simulink model "Model_01"  (R2014a)
settings: Solver=ode45  StartTime=0.0  StopTime=10.0  RelTol=1e-3
model workspace: external: MATLAB File C:\Users\Iseberg\Documents\MATLAB\Init_Model_01.m (data not in the file)
values from neighbouring files (symbols this model uses):
  e_force_x = 0    [Init_Model_01.m]    (also in Init_Model_02_Simulink.m)
  e_force_y = 0    [Init_Model_01.m]    (also in Init_Model_02_Simulink.m)
  e_force_z = 0    [Init_Model_01.m]    (also in Init_Model_02_Simulink.m)
  ita = [0.12;0.05;-0.15;0.98]    [Init_Model_01.m]    (also in Init_Model_02_Simulink.m)
  J_k = J    [Init_Model_01.m]
  om_x_0 = 0    [Init_Model_01.m]    (also in Init_Model_02_Simulink.m)
  om_y_0 = 0    [Init_Model_01.m]    (also in Init_Model_02_Simulink.m)
  om_z_0 = 0    [Init_Model_01.m]    (also in Init_Model_02_Simulink.m)
  p_x = (i_yy - i_zz)/i_xx    (= 0.75)    [Init_Model_01.m]    (also in Init_Model_02_Simulink.m)
  p_x_0 = p_x    (= 0.75)    [Init_Model_01.m]    (also in Init_Model_02_Simulink.m = 2)
  p_y = (i_zz - i_xx)/i_yy    (= 0.125)    [Init_Model_01.m]    (also in Init_Model_02_Simulink.m)
  p_y_0 = p_y    (= 0.125)    [Init_Model_01.m]    (also in Init_Model_02_Simulink.m = -0.5)
  p_z = (i_xx - i_yy)/i_zz    (= -0.8)    [Init_Model_01.m]    (also in Init_Model_02_Simulink.m)
  p_z_0 = p_z    (= -0.8)    [Init_Model_01.m]    (also in Init_Model_02_Simulink.m = -2)
  q_0_0 = 1    [Init_Model_01.m]    (also in Init_Model_02_Simulink.m)
  q_1_0 = 0    [Init_Model_01.m]    (also in Init_Model_02_Simulink.m)
  q_2_0 = 0    [Init_Model_01.m]    (also in Init_Model_02_Simulink.m)
  q_3_0 = 0    [Init_Model_01.m]    (also in Init_Model_02_Simulink.m)
  r_dot_x_0 = 0    [Init_Model_01.m]    (also in Init_Model_02_Simulink.m)
  r_dot_y_0 = 0    [Init_Model_01.m]    (also in Init_Model_02_Simulink.m)
  r_dot_z_0 = 0    [Init_Model_01.m]    (also in Init_Model_02_Simulink.m)
  r_x_0 = 0    [Init_Model_01.m]    (also in Init_Model_02_Simulink.m)
  r_y_0 = 0    [Init_Model_01.m]    (also in Init_Model_02_Simulink.m)
  r_z_0 = 0    [Init_Model_01.m]    (also in Init_Model_02_Simulink.m)
  rho = [0.2;0.1;0.05]    [Init_Model_01.m]    (also in Init_Model_02_Simulink.m; quatErrorTest.m = fn_CrossTensor([a_g;2],0)*q_ref)
  sig_p = 1e-4    (= 0.0001)    [Init_Model_01.m]    (also in Init_Model_02_Simulink.m)
  sig_tau = 2.5e-5    (= 2.5e-05)    [Init_Model_01.m]    (also in Init_Model_02_Simulink.m)
  sig_theta = 1e-4    (= 0.0001)    [Init_Model_01.m]    (also in Init_Model_02_Simulink.m = 1e-06)
  tau_1 = 0    [Init_Model_01.m]    (also in Init_Model_02_Simulink.m)
  tau_2 = 0    [Init_Model_01.m]    (also in Init_Model_02_Simulink.m)
  tau_3 = 0    [Init_Model_01.m]    (also in Init_Model_02_Simulink.m)
undefined symbols (not defined in the file or in its folder): DiscIntNeverNeededParam
settings Model: Creator=Iseberg  LastModifiedBy=Iseberg

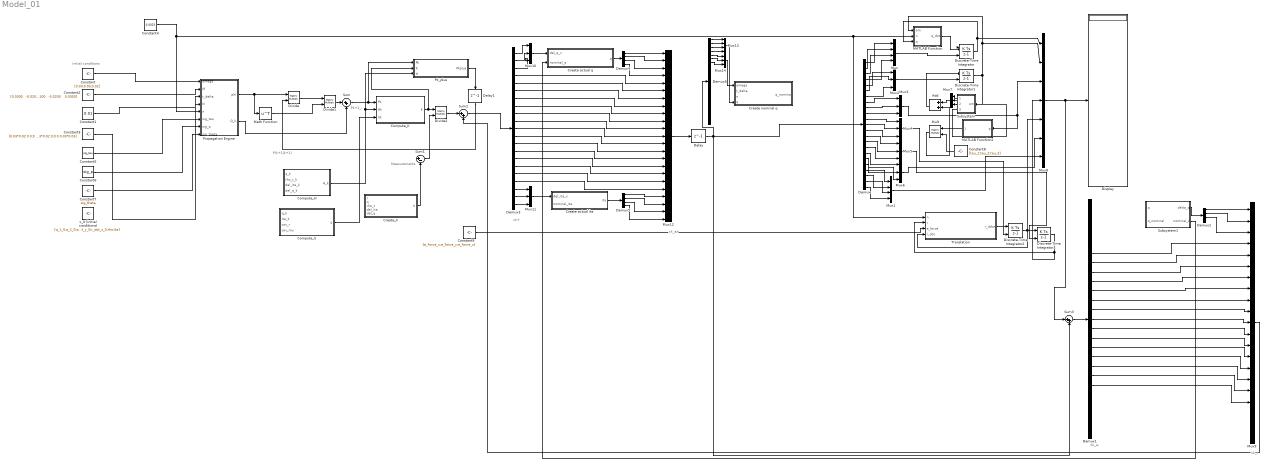
== system Model_01 ==
  note: initial conditions
  note: Pk+1_-
  note: xk_-
  note: xk_a-
  note: xk_a+
  note: xk+
  note: Measurements
  note: P(k+1|k+1)
  Add : Sum
  Compute_H : Subsystem
  Compute_K : MATLAB Function  TreatAsAtomicUnit=on
  Compute_S : MATLAB Function  TreatAsAtomicUnit=on
  Constant : Constant  Value=[0.03;0.03;0.02]
  Constant1 : Constant  Value=0.01
  Constant2 : Constant  Value="[0.0300   -0.0200    0.0100;-0.0200    0.0200   -0.0100;0.0100   -0.0200    0.0300]"
  Constant3 : Constant  Value=[0.03*0.02 0 0;0 0.03*0.02 0;0 0 0.03*0.03]
  Constant4 : Constant  Value=0.0023
  Constant5 : Constant  Value=sig_tau
  Constant6 : Constant  Value=sig_p
  Constant7 : Constant  Value=sig_theta
  Constant8 : Constant  Value=[tau_1;tau_2;tau_3]
  Constant9 : Constant  Value=[e_force_x;e_force_y;e_force_z]
  Create actual ita : MATLAB Function  TreatAsAtomicUnit=on
  Create actual q : MATLAB Function  TreatAsAtomicUnit=on
  Create nominal q : MATLAB Function  TreatAsAtomicUnit=on
  Create_h : MATLAB Function  TreatAsAtomicUnit=on
  Delay : Delay  DelayLength=1  InitialCondition=0
  Delay1 : Delay  DelayLength=1  InitialCondition=0
  Demux : Demux  Outputs=23
  Demux1 : Demux  Outputs=23
  Demux2 : Demux
  Demux3 : Demux  Outputs=21
  Demux4 : Demux
  Demux5 : Demux
  Demux6 : Demux  Outputs=23
  Discrete-Time Integrator{,1..3} (4 alike) : DiscreteIntegrator  InitialConditionSource=external  ICPrevOutput=DiscIntNeverNeededParam  ICPrevScaledInput=DiscIntNeverNeededParam
  Display : Display
  Divide : Product  Inputs=**  Multiplication=Matrix(*)
  Divide1 : Product  Inputs=**  Multiplication=Matrix(*)
  Divide2 : Product  Inputs=**  Multiplication=Matrix(*)
  MATLAB Function : MATLAB Function  TreatAsAtomicUnit=on
  MATLAB Function2 : MATLAB Function  TreatAsAtomicUnit=on
  Math Function : Math  Operator=transpose  SaturateOnIntegerOverflow=on
  Mult : Product  Inputs=**  Multiplication=Matrix(*)
  Mux : Mux
  Mux1 : Mux
  Mux{2..7,10..11,14} (9 alike) : Mux  Inputs=3
  Mux12 : Mux  Inputs=23
  Mux13 : Mux
  Mux8 : Mux  Inputs=7
  Mux9 : Mux  Inputs=21
  Pk_plus : MATLAB Function  TreatAsAtomicUnit=on
  Propagation Engine : Subsystem
  Subsystem : Subsystem
  Subsystem1 : Subsystem
  Sum : Sum  Inputs=|++
  Sum1 : Sum  Inputs=|+-
  Sum2 : Sum  Inputs=|++
  Sum3 : Sum  Inputs=|++
  Translation : MATLAB Function  TreatAsAtomicUnit=on
  x_0 (initial conditions) : Constant  Value=[q_1_0;q_2_0;q_3_0;q_0_0;om_x_0;om_y_0;om_z_0;p_x_0;p_y_0;p_z_0;r_x_0;r_y_0;r_z_0;r_dot_x_0;r_dot_y_0;r_dot_z_0;rho;ita]  VectorParams1D=off
  wires:
  Constant/1 -> Propagation Engine/1(omega)
  Constant2/1 -> Propagation Engine/2(M)
  Constant1/1 -> Propagation Engine/3(t_delta)
  Constant3/1 -> Propagation Engine/4(N)
  Constant4/1 -> Propagation Engine/5(n), Translation/1(n), MATLAB Function/2(n)
  Constant5/1 -> Propagation Engine/6(sig_tau)
  Constant6/1 -> Propagation Engine/7(sig_p)
  Demux/1 -> Mux/1
  Demux/2 -> Mux/2
  Demux/3 -> Mux/3
  Demux/4 -> Mux/4
  Demux/20 -> Mux1/1
  Demux/21 -> Mux1/2
  Demux/22 -> Mux1/3
  Demux/23 -> Mux1/4
  Demux/5 -> Mux2/1
  Demux/6 -> Mux2/2
  Demux/7 -> Mux2/3
  Demux/8 -> Mux3/1
  Demux/9 -> Mux3/2
  Demux/10 -> Mux3/3
  Demux/11 -> Mux4/1
  Demux/12 -> Mux4/2
  Demux/13 -> Mux4/3
  Demux/14 -> Mux5/1
  Demux/15 -> Mux5/2
  Demux/16 -> Mux5/3
  Demux/17 -> Mux6/1
  Demux/18 -> Mux6/2
  Demux/19 -> Mux6/3
  Mux/1 -> Discrete-Time Integrator/2
  MATLAB Function/1(q_dot) -> Discrete-Time Integrator/1
  Discrete-Time Integrator/1 -> Mux8/1, MATLAB Function/3(q)
  Mux2/1 -> Discrete-Time Integrator1/2
  Discrete-Time Integrator1/1 -> Subsystem/1(om), Mux8/2, MATLAB Function/1(om)
  Constant8/1 -> Mult/2
  Mult/1 -> Add/2
  Subsystem/1(psi_1) -> Mux7/1
  Subsystem/2(psi_2) -> Mux7/2
  Subsystem/3("psi_3 ") -> Mux7/3
  Mux7/1 -> Add/1
  Add/1 -> Discrete-Time Integrator1/1
  Translation/1(r_ddot) -> Discrete-Time Integrator2/1
  Constant9/1 -> Translation/3(e_force)
  Mux4/1 -> Discrete-Time Integrator2/2
  Mux5/1 -> Discrete-Time Integrator3/2
  Mux3/1 -> Mux8/3, MATLAB Function2/1(p)
  Discrete-Time Integrator3/1 -> Mux8/4, Translation/2(r)
  Discrete-Time Integrator2/1 -> Discrete-Time Integrator3/1, Mux8/5, Translation/4(r_dot)
  Mux6/1 -> Mux8/6
  Mux1/1 -> Mux8/7
  MATLAB Function2/1(J) -> Mult/1
  Mux8/1 -> Sum3/1, Display/1
  Constant7/1 -> Propagation Engine/8(sig_theta)
  Propagation Engine/1("phi ") -> Math Function/1, Divide/1
  Divide/1 -> Divide1/1
  Math Function/1 -> Divide1/2
  Divide1/1 -> Sum/1
  Propagation Engine/2("Q_k ") -> Sum/2
  Sum/1 -> Compute_K/1(Pk), Pk_plus/1(Pk)
  Compute_H/1(H_k) -> Pk_plus/3(H), Compute_K/2(Hk)
  Compute_K/1(K) -> Pk_plus/2(K), Divide2/1
  Sum1/1 -> Divide2/2
  Divide2/1 -> Sum2/1
  Create_h/1(h) -> Sum1/2
  ? -> Sum1/1
  Subsystem1/1(delta_q) -> Demux2/1
  Demux2/1 -> Mux9/1
  Demux2/2 -> Mux9/2
  Demux2/3 -> Mux9/3
  Demux1/5 -> Mux9/4
  Demux1/6 -> Mux9/5
  Demux1/7 -> Mux9/6
  Demux1/8 -> Mux9/7
  Demux1/9 -> Mux9/8
  Demux1/10 -> Mux9/9
  Demux1/11 -> Mux9/10
  Demux1/12 -> Mux9/11
  Demux1/13 -> Mux9/12
  Demux1/14 -> Mux9/13
  Demux1/15 -> Mux9/14
  Demux1/16 -> Mux9/15
  Demux1/17 -> Mux9/16
  Demux1/18 -> Mux9/17
  Demux1/19 -> Mux9/18
  Mux9/1 -> Sum2/2
  Compute_S/1(S) -> Compute_K/3(Sk)
  Sum2/1 -> Demux3/1
  Subsystem1/2(nominal_q) -> Create actual q/2(nominal_q)
  Demux3/1 -> Mux10/1
  Demux3/2 -> Mux10/2
  Demux3/3 -> Mux10/3
  Mux10/1 -> Create actual q/1(del_q_v)
  Mux11/1 -> Create actual ita/1(del_ita_v)
  Demux3/19 -> Mux11/1
  Demux3/20 -> Mux11/2
  Demux3/21 -> Mux11/3
  Create actual q/1(q) -> Demux4/1
  Create actual ita/1(ita) -> Demux5/1
  Demux4/1 -> Mux12/1
  Demux4/2 -> Mux12/2
  Demux4/3 -> Mux12/3
  Demux4/4 -> Mux12/4
  Demux3/4 -> Mux12/5
  Demux3/5 -> Mux12/6
  Demux3/6 -> Mux12/7
  Demux3/7 -> Mux12/8
  Demux3/8 -> Mux12/9
  Demux3/9 -> Mux12/10
  Demux3/10 -> Mux12/11
  Demux3/11 -> Mux12/12
  Demux3/12 -> Mux12/13
  Demux3/13 -> Mux12/14
  Demux3/14 -> Mux12/15
  Demux3/15 -> Mux12/16
  Demux3/16 -> Mux12/17
  Demux3/17 -> Mux12/18
  Demux3/18 -> Mux12/19
  Demux5/1 -> Mux12/20
  Demux5/2 -> Mux12/21
  Demux5/3 -> Mux12/22
  Demux5/4 -> Mux12/23
  Sum3/1 -> Demux1/1
  Mux12/1 -> Delay/1
  Delay/1 -> Sum3/2, Demux6/1, Demux/1
  Pk_plus/1(Pkplus) -> Delay1/1
  Delay1/1 -> Divide/2
  Demux6/1 -> Mux13/1
  Demux6/2 -> Mux13/2
  Demux6/3 -> Mux13/3
  Demux6/4 -> Mux13/4
  Mux13/1 -> Create nominal q/4(q)
  Demux6/5 -> Mux14/1
  Demux6/6 -> Mux14/2
  Demux6/7 -> Mux14/3
  Mux14/1 -> Create nominal q/1(omega)

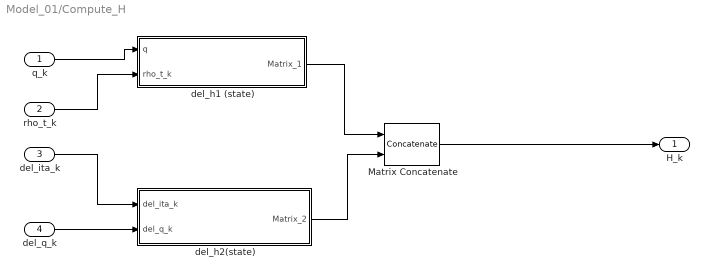
== system Model_01/Compute_H ==
  q_k : Inport
  rho_t_k : Inport  Port=2
  del_ita_k : Inport  Port=3
  del_q_k : Inport  Port=4
  Matrix Concatenate : Concatenate  Mode=Multidimensional array
  del_h1 (state) : MATLAB Function  TreatAsAtomicUnit=on
  del_h2(state) : MATLAB Function  TreatAsAtomicUnit=on
  H_k : Outport
  wires:
  q_k/1 -> del_h1 (state)/1(q)
  rho_t_k/1 -> del_h1 (state)/2(rho_t_k)
  del_ita_k/1 -> del_h2(state)/1(del_ita_k)
  del_q_k/1 -> del_h2(state)/2(del_q_k)
  del_h1 (state)/1(Matrix_1) -> Matrix Concatenate/1
  del_h2(state)/1(Matrix_2) -> Matrix Concatenate/2
  Matrix Concatenate/1 -> H_k/1

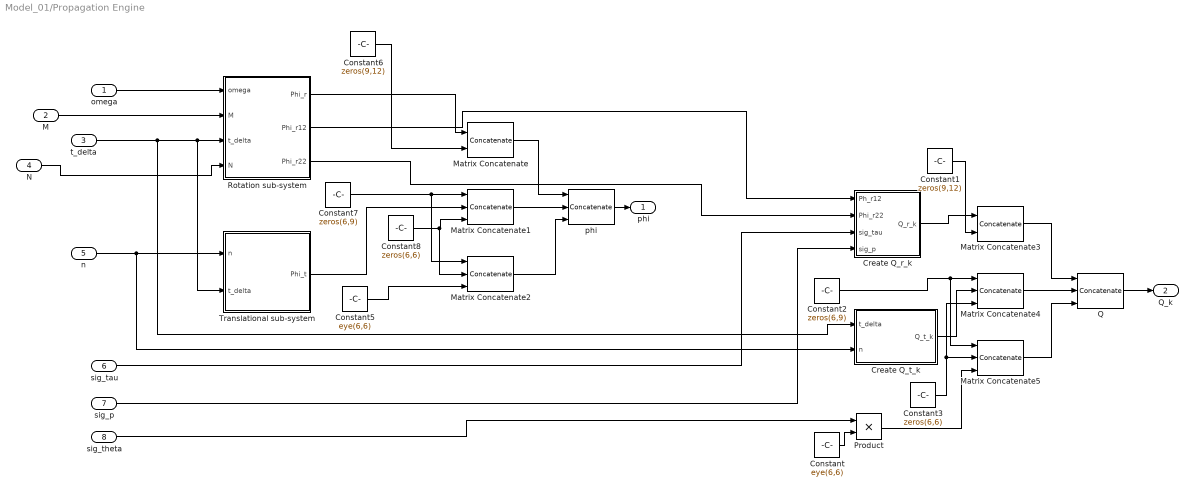
== system Model_01/Propagation Engine ==
  omega : Inport
  M : Inport  Port=2
  t_delta : Inport  Port=3
  N : Inport  Port=4
  n : Inport  Port=5
  sig_tau : Inport  Port=6
  sig_p : Inport  Port=7
  sig_theta : Inport  Port=8
  Constant : Constant  Value=eye(6,6)
  Constant1 : Constant  Value=zeros(9,12)  VectorParams1D=off
  Constant2 : Constant  Value=zeros(6,9)  VectorParams1D=off
  Constant3 : Constant  Value=zeros(6,6)  VectorParams1D=off
  Constant5 : Constant  Value=eye(6,6)  VectorParams1D=off
  Constant6 : Constant  Value=zeros(9,12)  VectorParams1D=off
  Constant7 : Constant  Value=zeros(6,9)  VectorParams1D=off
  Constant8 : Constant  Value=zeros(6,6)  VectorParams1D=off
  Create Q_r_k : Subsystem
  Create Q_t_k : MATLAB Function  TreatAsAtomicUnit=on
  Matrix Concatenate : Concatenate  Mode=Multidimensional array  ConcatenateDimension=2
  Matrix Concatenate{1..2,4..5} (4 alike) : Concatenate  NumInputs=3  Mode=Multidimensional array  ConcatenateDimension=2
  Matrix Concatenate3 : Concatenate  Mode=Multidimensional array  ConcatenateDimension=2
  Product : Product
  Q : Concatenate  NumInputs=3  Mode=Multidimensional array
  Rotation sub-system : Subsystem
  Translational sub-system : MATLAB Function  TreatAsAtomicUnit=on
  phi : Concatenate  NumInputs=3  Mode=Multidimensional array
  "phi " : Outport
  "Q_k " : Outport  Port=2
  wires:
  omega/1 -> Rotation sub-system/1(omega)
  M/1 -> Rotation sub-system/2(M)
  t_delta/1 -> Create Q_t_k/1(t_delta), Translational sub-system/2(t_delta), Rotation sub-system/3(t_delta)
  N/1 -> Rotation sub-system/4(N)
  n/1 -> Create Q_t_k/2(n), Translational sub-system/1(n)
  Rotation sub-system/1("Phi_r ") -> Matrix Concatenate/1
  Constant6/1 -> Matrix Concatenate/2
  Translational sub-system/1(Phi_t) -> Matrix Concatenate1/2
  Matrix Concatenate/1 -> phi/1
  Matrix Concatenate1/1 -> phi/2
  Matrix Concatenate2/1 -> phi/3
  Constant7/1 -> Matrix Concatenate2/1, Matrix Concatenate1/1
  Constant8/1 -> Matrix Concatenate2/2, Matrix Concatenate1/3
  phi/1 -> "phi "/1
  Constant5/1 -> Matrix Concatenate2/3
  Rotation sub-system/2(Phi_r12) -> Create Q_r_k/1("Ph_r12 ")
  Rotation sub-system/3(Phi_r22) -> Create Q_r_k/2(Phi_r22)
  sig_tau/1 -> Create Q_r_k/3(sig_tau)
  sig_p/1 -> Create Q_r_k/4(sig_p)
  Constant/1 -> Product/2
  sig_theta/1 -> Product/1
  Create Q_r_k/1(Q_r_k) -> Matrix Concatenate3/1
  Constant1/1 -> Matrix Concatenate3/2
  Create Q_t_k/1(Q_t_k) -> Matrix Concatenate4/2
  Constant2/1 -> Matrix Concatenate5/1, Matrix Concatenate4/1
  Constant3/1 -> Matrix Concatenate5/2, Matrix Concatenate4/3
  Product/1 -> Matrix Concatenate5/3
  Matrix Concatenate3/1 -> Q/1
  Matrix Concatenate4/1 -> Q/2
  Matrix Concatenate5/1 -> Q/3
  Q/1 -> "Q_k "/1

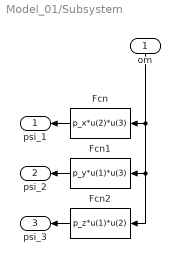
== system Model_01/Subsystem ==
  om : Inport
  Fcn : Fcn  Expr=p_x*u(2)*u(3)
  Fcn1 : Fcn  Expr=p_y*u(1)*u(3)
  Fcn2 : Fcn  Expr=p_z*u(1)*u(2)
  psi_1 : Outport
  psi_2 : Outport  Port=2
  "psi_3 " : Outport  Port=3
  wires:
  Fcn/1 -> psi_1/1
  Fcn2/1 -> "psi_3 "/1
  om/1 -> Fcn2/1, Fcn1/1, Fcn/1
  Fcn1/1 -> psi_2/1

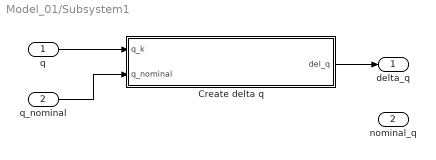
== system Model_01/Subsystem1 ==
  q : Inport
  "q_nominal " : Inport  Port=2
  Create delta q : MATLAB Function  TreatAsAtomicUnit=on
  delta_q : Outport
  nominal_q : Outport  Port=2
  wires:
  q/1 -> Create delta q/1(q_k)
  Create delta q/1(del_q) -> delta_q/1
  "q_nominal "/1 -> Create delta q/2(q_nominal)

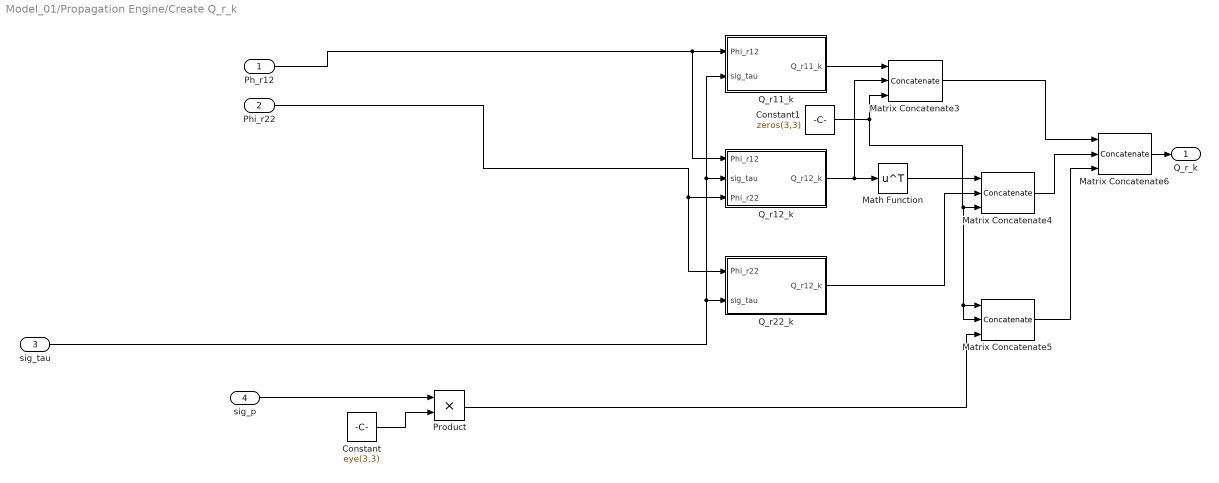
== system Model_01/Propagation Engine/Create Q_r_k ==
  "Ph_r12 " : Inport
  Phi_r22 : Inport  Port=2
  sig_tau : Inport  Port=3
  sig_p : Inport  Port=4
  Constant : Constant  Value=eye(3,3)
  Constant1 : Constant  Value=zeros(3,3)  VectorParams1D=off
  Math Function : Math  Operator=transpose  SaturateOnIntegerOverflow=on
  Matrix Concatenate3 : Concatenate  NumInputs=3  Mode=Multidimensional array  ConcatenateDimension=2
  Matrix Concatenate4 : Concatenate  NumInputs=3  Mode=Multidimensional array  ConcatenateDimension=2
  Matrix Concatenate5 : Concatenate  NumInputs=3  Mode=Multidimensional array  ConcatenateDimension=2
  Matrix Concatenate6 : Concatenate  NumInputs=3  Mode=Multidimensional array
  Product : Product
  Q_r11_k : Subsystem
  Q_r12_k : Subsystem
  Q_r22_k : Subsystem
  Q_r_k : Outport
  wires:
  Matrix Concatenate5/1 -> Matrix Concatenate6/3
  Matrix Concatenate3/1 -> Matrix Concatenate6/1
  Matrix Concatenate4/1 -> Matrix Concatenate6/2
  Q_r22_k/1(Q_r12_k) -> Matrix Concatenate4/2
  Math Function/1 -> Matrix Concatenate4/1
  Phi_r22/1 -> Q_r22_k/1(Phi_r22), Q_r12_k/3(Phi_r22)
  "Ph_r12 "/1 -> Q_r12_k/1(Phi_r12), Q_r11_k/1(Phi_r12)
  sig_tau/1 -> Q_r22_k/2("sig_tau "), Q_r12_k/2("sig_tau "), Q_r11_k/2("sig_tau ")
  Constant1/1 -> Matrix Concatenate5/2, Matrix Concatenate5/1, Matrix Concatenate4/3, Matrix Concatenate3/3
  Matrix Concatenate6/1 -> Q_r_k/1
  Q_r11_k/1(Q_r11_k) -> Matrix Concatenate3/1
  Q_r12_k/1(Q_r12_k) -> Math Function/1, Matrix Concatenate3/2
  sig_p/1 -> Product/1
  Constant/1 -> Product/2
  Product/1 -> Matrix Concatenate5/3

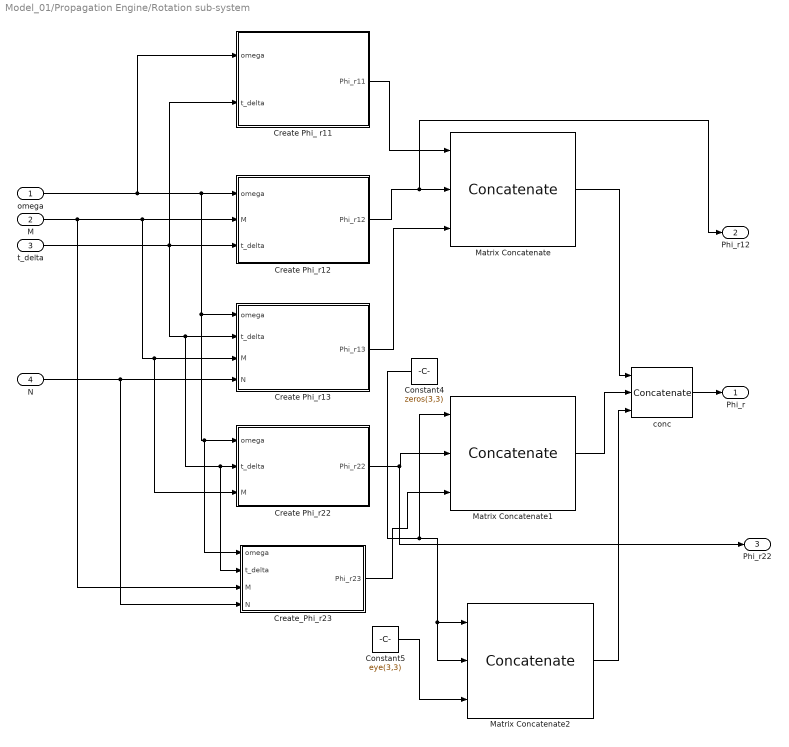
== system Model_01/Propagation Engine/Rotation sub-system ==
  omega : Inport
  M : Inport  Port=2
  t_delta : Inport  Port=3
  N : Inport  Port=4
  Constant4 : Constant  Value=zeros(3,3)
  Constant5 : Constant  Value=eye(3,3)
  "Create Phi_ r11 " : MATLAB Function  TreatAsAtomicUnit=on
  "Create Phi_r12 " : MATLAB Function  TreatAsAtomicUnit=on
  "Create Phi_r13 " : MATLAB Function  TreatAsAtomicUnit=on
  Create Phi_r22 : MATLAB Function  TreatAsAtomicUnit=on
  Create_Phi_r23 : MATLAB Function  TreatAsAtomicUnit=on
  Matrix Concatenate : Concatenate  NumInputs=3  Mode=Multidimensional array  ConcatenateDimension=2
  Matrix Concatenate1 : Concatenate  NumInputs=3  Mode=Multidimensional array  ConcatenateDimension=2
  Matrix Concatenate2 : Concatenate  NumInputs=3  Mode=Multidimensional array  ConcatenateDimension=2
  conc : Concatenate  NumInputs=3  Mode=Multidimensional array
  "Phi_r " : Outport
  Phi_r12 : Outport  Port=2
  Phi_r22 : Outport  Port=3
  wires:
  omega/1 -> "Create Phi_ r11 "/1(omega), Create_Phi_r23/1(omega), Create Phi_r22/1(omega), "Create Phi_r13 "/1(omega), "Create Phi_r12 "/1(omega)
  t_delta/1 -> Create_Phi_r23/2(t_delta), Create Phi_r22/2(t_delta), "Create Phi_r13 "/2(t_delta), "Create Phi_ r11 "/2(t_delta), "Create Phi_r12 "/3(t_delta)
  M/1 -> Create_Phi_r23/3(M), Create Phi_r22/3(M), "Create Phi_r13 "/3(M), "Create Phi_r12 "/2(M)
  "Create Phi_r12 "/1(Phi_r12) -> Phi_r12/1, Matrix Concatenate/2
  "Create Phi_ r11 "/1(Phi_r11) -> Matrix Concatenate/1
  N/1 -> Create_Phi_r23/4(N), "Create Phi_r13 "/4(N)
  "Create Phi_r13 "/1(Phi_r13) -> Matrix Concatenate/3
  Create_Phi_r23/1(Phi_r23) -> Matrix Concatenate1/3
  Matrix Concatenate2/1 -> conc/3
  Matrix Concatenate/1 -> conc/1
  Constant4/1 -> Matrix Concatenate1/1, Matrix Concatenate2/2, Matrix Concatenate2/1
  Create Phi_r22/1(Phi_r22) -> Phi_r22/1, Matrix Concatenate1/2
  Matrix Concatenate1/1 -> conc/2
  Constant5/1 -> Matrix Concatenate2/3
  conc/1 -> "Phi_r "/1

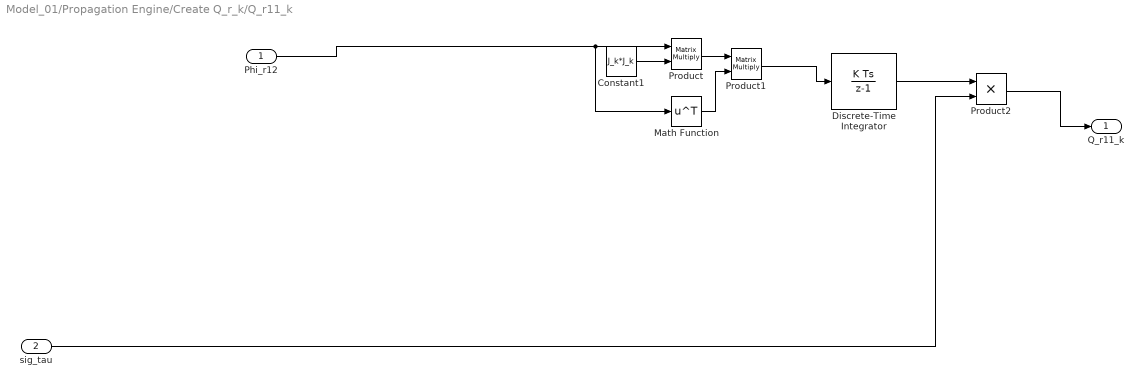
== system Model_01/Propagation Engine/Create Q_r_k/Q_r11_k ==
  Phi_r12 : Inport
  "sig_tau " : Inport  Port=2
  Constant1 : Constant  Value=J_k*J_k  VectorParams1D=off
  Discrete-Time Integrator : DiscreteIntegrator  ICPrevOutput=DiscIntNeverNeededParam  ICPrevScaledInput=DiscIntNeverNeededParam
  Math Function : Math  Operator=transpose  SaturateOnIntegerOverflow=on
  Product : Product  Multiplication=Matrix(*)
  Product1 : Product  Multiplication=Matrix(*)
  Product2 : Product
  Q_r11_k : Outport
  wires:
  Product/1 -> Product1/1
  Constant1/1 -> Product/2
  Product1/1 -> Discrete-Time Integrator/1
  Discrete-Time Integrator/1 -> Product2/1
  "sig_tau "/1 -> Product2/2
  Product2/1 -> Q_r11_k/1
  Math Function/1 -> Product1/2
  Phi_r12/1 -> Product/1, Math Function/1

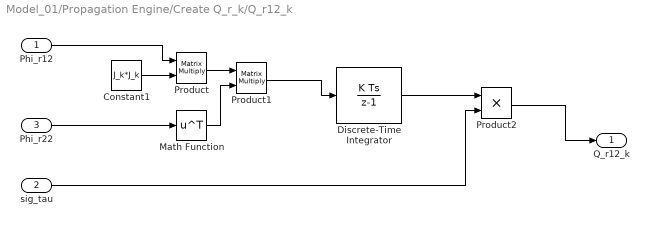
== system Model_01/Propagation Engine/Create Q_r_k/Q_r12_k ==
  Phi_r12 : Inport
  "sig_tau " : Inport  Port=2
  Phi_r22 : Inport  Port=3
  Constant1 : Constant  Value=J_k*J_k  VectorParams1D=off
  Discrete-Time Integrator : DiscreteIntegrator  ICPrevOutput=DiscIntNeverNeededParam  ICPrevScaledInput=DiscIntNeverNeededParam
  Math Function : Math  Operator=transpose  SaturateOnIntegerOverflow=on
  Product : Product  Multiplication=Matrix(*)
  Product1 : Product  Multiplication=Matrix(*)
  Product2 : Product
  Q_r12_k : Outport
  wires:
  Phi_r12/1 -> Product/1
  Math Function/1 -> Product1/2
  Product2/1 -> Q_r12_k/1
  "sig_tau "/1 -> Product2/2
  Discrete-Time Integrator/1 -> Product2/1
  Product1/1 -> Discrete-Time Integrator/1
  Constant1/1 -> Product/2
  Product/1 -> Product1/1
  Phi_r22/1 -> Math Function/1

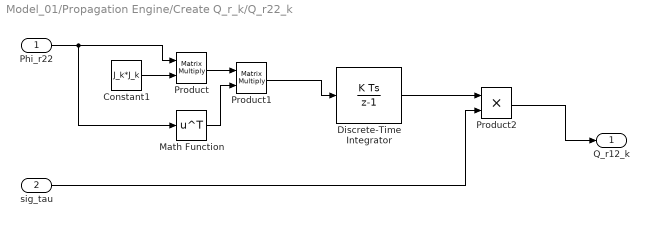
== system Model_01/Propagation Engine/Create Q_r_k/Q_r22_k ==
  Phi_r22 : Inport
  "sig_tau " : Inport  Port=2
  Constant1 : Constant  Value=J_k*J_k  VectorParams1D=off
  Discrete-Time Integrator : DiscreteIntegrator  ICPrevOutput=DiscIntNeverNeededParam  ICPrevScaledInput=DiscIntNeverNeededParam
  Math Function : Math  Operator=transpose  SaturateOnIntegerOverflow=on
  Product : Product  Multiplication=Matrix(*)
  Product1 : Product  Multiplication=Matrix(*)
  Product2 : Product
  Q_r12_k : Outport
  wires:
  Phi_r22/1 -> Math Function/1, Product/1
  Product/1 -> Product1/1
  Constant1/1 -> Product/2
  Product1/1 -> Discrete-Time Integrator/1
  Discrete-Time Integrator/1 -> Product2/1
  "sig_tau "/1 -> Product2/2
  Product2/1 -> Q_r12_k/1
  Math Function/1 -> Product1/2

== matlab function Model_01/Propagation Engine/Rotation sub-system/Create Phi_r12  ==
  data: omega input; Phi_r12 output; M input; t_delta input
function Phi_r12  = fn_Create_phi_r12(omega,M,t_delta)
%#codegen
    Phi_r12 = zeros(3,3);
    v_lambda = real(eig(M));
    %Set up matrix to solve for Gamma
    A = [1 v_lambda(1) v_lambda(1)^2;1 v_lambda(2) v_lambda(2)^2;1 v_lambda(3) v_lambda(3)^2];
    Gamma = real(inv(A));
    Omega_Tensor = fn_VectorToSkewSymmetricTensor(omega);
    omega_norm = norm(omega);
    for l=1:3
        for j=1:3
            for k= 1:3
                Phi_r12 = Phi_r12 + Gamma(l,j)*fn_phi_jk(k,v_lambda(j),t_delta, omega_norm)*(Omega_Tensor^(k-1))*(M^(l-1));
            end
        end
    end
    Phi_r12 = 0.5*Phi_r12;
end   

function phi_jk = fn_phi_jk(k,lambda,t_delta,omega_norm)
    switch(k)
        case 1
            phi_jk = fn_phi_j1(lambda,t_delta);
        case 2
            phi_jk = fn_phi_j2(lambda, omega_norm,t_delta);
        case 3
            phi_jk = fn_phi_j3(lambda, omega_norm, t_delta);
        otherwise
            phi_jk = 0;
    end
end

%Following functions are for jth lambda
function phi_j1 = fn_phi_j1(lambda,t_delta)    
    phi_j1 = (lambda^-1)*(exp(lambda*t_delta) - 1);
end
function phi_j2 = fn_phi_j2(lambda, omega_norm, t_delta)
    phi_j2 = ((lambda^2*omega_norm + omega_norm^3)^-1)*(omega_norm*cos(omega_norm*t_delta) + lambda*sin(omega_norm*t_delta) - exp(lambda*t_delta)*omega_norm);
end
function phi_j3 = fn_phi_j3(lambda, omega_norm, t_delta)
    phi_j3 = (omega_norm^-2)*(lambda^-1) + (lambda^3*omega_norm^2 + lambda*omega_norm^4)*((lambda^2)*cos(omega_norm*t_delta) - omega_norm*lambda*sin(omega_norm*t_delta) + (omega_norm^2)*exp(omega_norm*t_delta));
end

== matlab function Model_01/Propagation Engine/Rotation sub-system/Create Phi_ r11  ==
  data: omega input; Phi_r11 output; t_delta input
%Create the State Transition Matrix 11 for rotation kinematics
%Inputs: omega: angular velocity vector in current time step
%        t_delta: sampling time.
function Phi_r11 = fn_Create_phi_r11(omega, t_delta)
%#codegen
    Omega_Tensor = fn_VectorToSkewSymmetricTensor(omega);
    omega_norm = norm(omega);
    Phi_r11 = eye(3,3) - (sin(omega_norm*t_delta)/omega_norm)*Omega_Tensor + ((1-cos(omega_norm*t_delta))/omega_norm^2)*Omega_Tensor^2;
end

== matlab function Model_01/Propagation Engine/Rotation sub-system/Create Phi_r13  ==
  data: omega input; Phi_r13 output; t_delta input; M input; N input
function Phi_r13 = fn_Create_phi_r13(omega, t_delta,M,N)
%#codegen
    Phi_r13 = zeros(3,3);
    v_lambda = real(eig(M));
    A = [1 v_lambda(1) v_lambda(1)^2;1 v_lambda(2) v_lambda(2)^2;1 v_lambda(3) v_lambda(3)^2];
    Gamma = real(inv(A));
    for i = 1:3
        for j = 1:3
            Phi_r13 = Phi_r13 + Gamma(i,j)*(v_lambda(j)^-1)*(exp(v_lambda(j)*t_delta)-1)*(M^(i-1))*N;
        end
    end
end

== matlab function Model_01/Propagation Engine/Rotation sub-system/Create Phi_r22 ==
  data: omega input; Phi_r22 output; t_delta input; M input
function Phi_r22 = fn_Create_phi_r22(omega,t_delta,M)
%#codegen
    Phi_r22 = zeros(3,3);
    v_lambda = real(eig(M));
    A = [1 v_lambda(1) v_lambda(1)^2;1 v_lambda(2) v_lambda(2)^2;1 v_lambda(3) v_lambda(3)^2];
    Gamma = real(inv(A));
    for i = 1:3
        for j = 1:3
            Phi_r22 = Phi_r22 + Gamma(i,j)*exp(v_lambda(j)*t_delta)*M^(i-1);
        end
    end
end

== matlab function Model_01/Propagation Engine/Rotation sub-system/Create_Phi_r23 ==
  data: omega input; Phi_r23 output; t_delta input; M input; N input
function Phi_r23 = fn_Create_phi_r23(omega, t_delta, M, N)
%#codegen
    Phi_r23 = zeros(3,3);
    Omega_Tensor = fn_VectorToSkewSymmetricTensor(omega);
    omega_norm = norm(omega);
    v_lambda = real(eig(M));
    A = [1 v_lambda(1) v_lambda(1)^2;1 v_lambda(2) v_lambda(2)^2;1 v_lambda(3) v_lambda(3)^2];
    Gamma = real(inv(A));
    for i= 1:3
        for j = 1:3
            for k = 1:3
                Phi_r23 = Phi_r23 + Gamma(i,j)*fn_phi_jk(k,v_lambda(j),omega_norm,t_delta)*(Omega_Tensor^(k-1))*(M^(i-1))*N;
            end
        end
    end
end
function phi_jk = fn_phi_jk(k,lambda,omega_norm,t_delta)
    switch(k)
        case 1
            phi_jk = fn_phi_j1(lambda, t_delta);
        case 2
            phi_jk = fn_phi_j2(lambda, omega_norm,t_delta);
        case 3
            phi_jk = fn_phi_j3(lambda, omega_norm, t_delta);
        otherwise
            phi_jk = 0;
    end
end

function phi_j1 = fn_phi_j1(lambda, t_delta)
    phi_j1 = (lambda^-2)*(1-exp(lambda*t_delta)) - (lambda^-1)*t_delta;
end

function phi_j2 = fn_phi_j2(lambda, omega_norm, t_delta)
    phi_j2 = ((lambda^3)*(omega_norm^2) + (lambda*(omega_norm^4))^-1)*(omega_norm*lambda*sin(omega_norm*t_delta) + (lambda^2)*cos(omega_norm*t_delta) + (omega_norm^2)*exp(omega_norm*t_delta) - lambda^2 - omega_norm^2);
end
    
function phi_j3 = fn_phi_j3(lambda, omega_norm, t_delta)
    phi_j3 = (omega_norm^-2)*(lambda^-2) + (((lambda^4)*(omega_norm^3) + (lambda^2)*(omega_norm^5))^-1)*((lambda^3)*sin(omega_norm*t_delta) - omega_norm*(lambda^2)*cos(omega_norm*t_delta) - (omega_norm^3)*exp(omega_norm*t_delta) - ((omega_norm^3)*lambda + (lambda^3)*omega_norm)*t_delta);
end

== matlab function Model_01/Propagation Engine/Translational sub-system ==
  data: n input; Phi_t output; t_delta input
function Phi_t = fn_Create_Phi_t(n,t_delta)
%#codegen
    Phi_t12 = [t_delta, n*t_delta^2,0;0, t_delta, 0;0,0,t_delta];
    Phi_t22 = eye(3,3) - 2*fn_VectorToSkewSymmetricTensor([0;0;n])*t_delta;
    
    Phi_t = [eye(3,3),Phi_t12;zeros(3,3),Phi_t22];
    
end

== matlab function Model_01/Propagation Engine/Create Q_t_k ==
  data: t_delta input; Q_t_k output; n input
function Q_t_k  = fn_Create_Q_t_k(t_delta, n)
%#codegen

Q_t11_k = [(t_delta^3)/3 + (2/5)*n^2*t_delta^5, (1/4)*(n - n^2)*t_delta^4, 0;(1/4)*(n - n^2)*t_delta^4, (t_delta^3)/3 - (4/15)*n^2*t_delta^5 0;0, 0, (t_delta^3)/3 - (1/15)*n^2*t_delta^5];
Q_t12_k = [(t_delta^2)/2 + (1/3)*(n^2)*(t_delta^4), -(1/3)*n*(t_delta^3),0;(2/3)*(n - n^2)*t_delta^3, (1/2)*(t_delta^2) - (2/3)*(n^2)*(t_delta^4) 0;0 0 (1/2)*(t_delta^2) - (1/6)*(n^2)*(t_delta^4)];
Q_t22_k = [t_delta + (n^2)*(t_delta^3), 0, 0;0, t_delta, 0;0, 0, t_delta - (1/3)*(n^2)*(t_delta^3)];

Q_t_k = [Q_t11_k, Q_t12_k;Q_t12_k',Q_t22_k];

end

== matlab function Model_01/MATLAB Function ==
  data: om input; q_dot output; n input; q input
function q_dot  = fn_Create_qdot(om, n, q)
    v_n = [0;0;n];
    q_n = [v_n;0];
    q_om = [om;0];
    Tensor_om = fn_CrossTensor(q_om,0);
    Tensor_n = fn_CrossTensor(q_n,1);
    q_dot = (1/2)*(Tensor_om - Tensor_n)*q;
end

== matlab function Model_01/Translation ==
  data: n input; r_ddot output; r input; e_force input; r_dot input
function r_ddot = fn_Compute_r_ddot(n,r,e_force,r_dot)
%#codegen
    parameter_gravitation = 398.6005e12;
    re = [(parameter_gravitation/n^2)^(1/3);0;0];
    v_n = [0;0;n];
    Tensor_n = fn_VectorToSkewSymmetricTensor(v_n);
    Term_1 = -2*Tensor_n*r_dot;
    Term_2 = Tensor_n*(Tensor_n*r);
    Term_3 = parameter_gravitation*(re + r)/(norm(re+r))^3;
    Term_4 = (n^2)*re;
    
    r_ddot = Term_1 - Term_2 - Term_3 + Term_4 + e_force;
end

== matlab function Model_01/MATLAB Function2 ==
  data: p input; J output
function J = fn_Create_J(p)
%#codegen
    J = [1,0,0;0, (1-p(2))/(1+p(1)), 0;0, 0, (1+p(3))/(1-p(1))];
end

== matlab function Model_01/Compute_H/del_h1 (state) ==
  data: q input; Matrix_1 output; rho_t_k input
function Matrix_1 = fn_Create_del_h1(q,rho_t_k)
%#codegen
    q_0 = q(4);
    q_v = q(1:3);
    Q_v = fn_VectorToSkewSymmetricTensor(q_v);
    R = (2*q_0^2 - 1)*eye(3,3) + 2*q_0*Q_v + 2*q_v*q_v';
    
    first = -2*R*fn_VectorToSkewSymmetricTensor(q_v)
    Matrix_1 = [first, zeros(3,6),eye(3,3),zeros(3,3),R,zeros(3,3)];
end

== matlab function Model_01/Compute_K ==
  data: Pk input; K output; Hk input; Sk input
function K = fn_ComputeKalmanGain(Pk,Hk,Sk)
%#codegen
    K = Pk*Hk'/(Hk*Pk*Hk' + Sk);
end

== matlab function Model_01/Compute_H/del_h2(state) ==
  data: del_ita_k input; Matrix_2 output; del_q_k input
function Matrix_2 = fn_Create_del_h2(del_ita_k,del_q_k)
%#codegen
    del_Ita_k = fn_VectorToSkewSymmetricTensor(del_ita_k);
    first = -del_Ita_k + del_ita_k(4)*eye(3,3);
    del_Q_k = fn_VectorToSkewSymmetricTensor(del_q_k) ;
    last = del_Q_k + del_q_k(4)*eye(3,3);
    
    Matrix_2 = [first, zeros(3,6),zeros(3,3),zeros(3,3),zeros(3,3),last];
end

== matlab function Model_01/Compute_S ==
  data: q_k input; S output; ita_k input; cov_r input; cov_mu input
function S   = fn_Create_S(q_k,ita_k,cov_r,cov_mu)
%#codegen
    Ita_Tensor = fn_CrossTensor(ita_k,0);
    Q_Tensor = fn_CrossTensor(q_k,1);
    T = [eye(3,3),zeros(3,1)]*Ita_Tensor*Q_Tensor;
    S = [cov_r,zeros(3,3);zeros(3,3), T*cov_mu*T'];
    

end

== matlab function Model_01/Create_h ==
  data: r input; h output; q input; rho_t input; del_ita input; del_q input
function h = fn_Create_h(r,q,rho_t,del_ita,del_q)
%#codegen
    q_0 = q(4);
    q_v = q(1:3);
    Q_v = fn_VectorToSkewSymmetricTensor(q_v);
    R_q = (2*q_0^2 - 1)*eye(3,3) + 2*q_0*Q_v + 2*q_v*q_v';
    h1 = r + R_q*rho_t;
    temp = fn_CrossTensor(del_ita,0)*del_q;
    h2 = temp(1:3);
    h = [h1;h2];    
end

== matlab function Model_01/Subsystem1/Create delta q ==
  data: q_k input; del_q output; q_nominal input
function del_q = fn_Create_q_variation(q_k,q_nominal)
%#codegen
    del_q = fn_CrossTensor(q_k,0)*q_nominal;    
end

== matlab function Model_01/Pk_plus ==
  data: Pk input; Pkplus output; K input; H input
function Pkplus = fn_Create_Pkplus(Pk,K,H)
%#codegen
    Pkplus = (eye(21,21) - K*H)*Pk;
end

== matlab function Model_01/Create actual q ==
  data: del_q_v input; q output; nominal_q input
function q = fn_Create_q(del_q_v,nominal_q)
%#codegen
    del_q_0 = sqrt(1-norm(q_v)^2);
    del_q = [del_q_v;del_q_0];
    Tensor_del_q = fn_CrossTensor(del_q,0);
    q = Tensor_del_q*nominal_q;
end

== matlab function Model_01/Create actual ita ==
  data: del_ita_v input; ita output; nominal_ita input
function ita = fn_Create_ita(del_ita_v,nominal_ita)
%#codegen
    del_ita_0 = sqrt(1-norm(del_ita_v)^2);
    del_ita = [del_ita_v;del_ita_0];
    Tensor_del_ita = fn_CrossTensor(del_ita,0);
    ita = Tensor_del_ita*nominal_ita;
end

== matlab function Model_01/Create nominal q ==
  data: omega input; q_nominal output; t_delta input; n input; q input
function q_nominal = fn_CreateNominal_q(omega,t_delta,n,q)
%#codegen
    omega_norm = norm(omega);
    c = cos(omega_norm*t_delta/2);
    s = sin(omega_norm*t_delta/2);
    exponential_first =( c + s )*eye(4,4);
    q_omega = [omega;0];
    q_n = [n;0];
    exponential_second = ((omega_norm*t_delta*c - 4*s)/(2*omega_norm))*fn_CrossTensor(q_omega,0);
    exponential_om = exponential_first - exponential_second;
    exponential_n = exp((1/2)*t_delta)*fn_CrossTensor(-q_n,1);
    exponential = exponential_om*exponential_n;
    q_nominal = exponential*q;

end
